simulink model "MAE547ComplianceControl"  (R2023b)
settings: Solver=VariableStepAuto  StartTime=0.0  StopTime=10  RelTol=1e-3
values from neighbouring files (symbols this model uses):
  Kd = diag([2 10 30 1 1 1])    [Parameters.m]
  Kp = diag([50 80 100 1 1 1])    [Parameters.m]
  l1 = param.l1    [B_Lagrangian.m]    (also in Manipulator.m = 0.4; Parameters.m)
  l2 = param.l2    [B_Lagrangian.m]    (also in Manipulator.m = 0.46; Parameters.m)
  l3 = param.l3    [B_Lagrangian.m]    (also in Manipulator.m = 0.15; Parameters.m)
  m1 = param.m1    [B_Lagrangian.m]    (also in Manipulator.m = 1)
  m2 = param.m2    [B_Lagrangian.m]    (also in Manipulator.m = 1)
  m3 = param.m3    [B_Lagrangian.m]    (also in Manipulator.m = 1)
  xd = Kinematics(q)    [Parameters.m]
undefined symbols (not defined in the file or in its folder): axis, wall
settings Model: Creator=andre  LastModifiedBy=zaner
settings SolverCC: AlgebraicLoopSolver=TrustRegion
settings DataIOCC: LimitDataPoints=on
settings DebuggingCC: UnconnectedInputMsg=warning  UnconnectedOutputMsg=warning  UnconnectedLineMsg=warning
settings ModelReferenceCC: EnableRefExpFcnMdlSchedulingChecks=on
settings RTWCC: DLArmComputeVersion=19.05

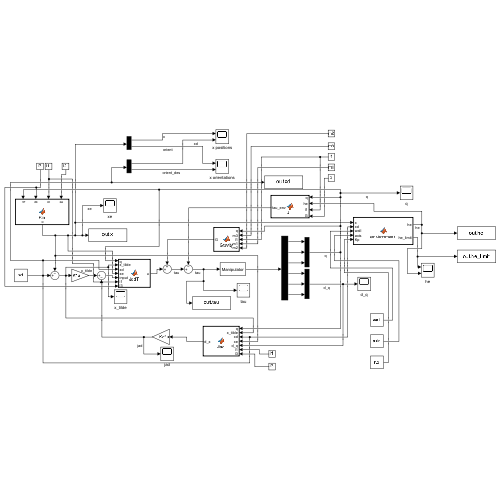
[thumbnail: Simulink's stored preview of the top-level diagram]
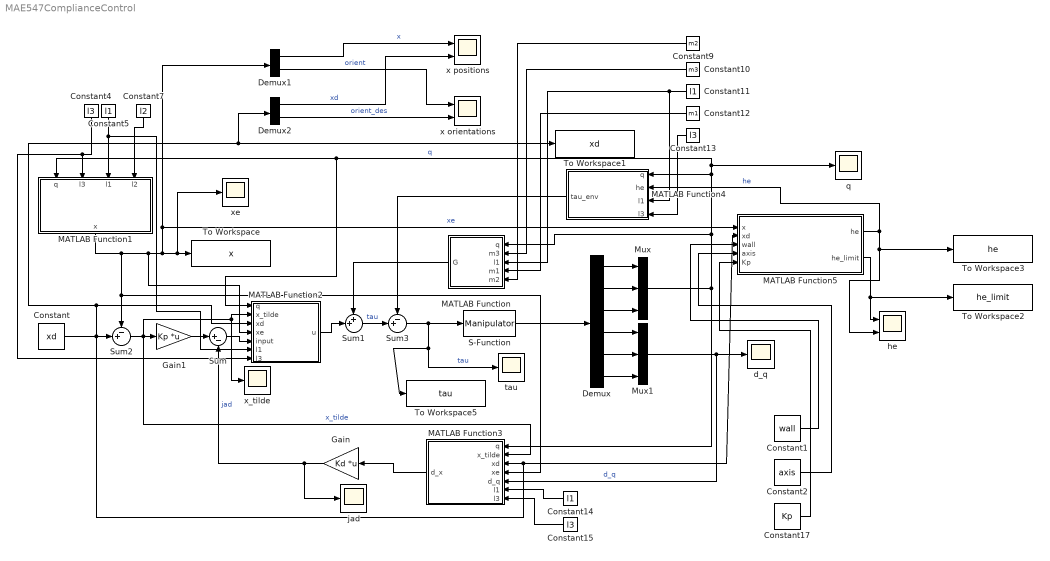
== system MAE547ComplianceControl ==
  Constant : Constant  Value=xd
  Constant1 : Constant  Value=wall
  Constant10 : Constant  Value=m3
  Constant11 : Constant  Value=l1
  Constant12 : Constant  Value=m1
  Constant13 : Constant  Value=l3
  Constant14 : Constant  Value=l1
  Constant15 : Constant  Value=l3
  Constant17 : Constant  Value=Kp
  Constant2 : Constant  Value=axis
  Constant4 : Constant  Value=l3
  Constant5 : Constant  Value=l1
  Constant7 : Constant  Value=l2
  Constant9 : Constant  Value=m2
  Demux : Demux  Outputs=6
  Demux1 : Demux  Outputs=2
  Demux2 : Demux  Outputs=2
  Gain : Gain  Gain=Kd  Multiplication=Matrix(K*u)
  Gain1 : Gain  Gain=Kp  Multiplication=Matrix(K*u)
  MATLAB Function : MATLAB Function  TreatAsAtomicUnit=on
  MATLAB Function1 : MATLAB Function  TreatAsAtomicUnit=on
  MATLAB Function2 : MATLAB Function  TreatAsAtomicUnit=on
  MATLAB Function3 : MATLAB Function  TreatAsAtomicUnit=on
  MATLAB Function4 : MATLAB Function  TreatAsAtomicUnit=on
  MATLAB Function5 : MATLAB Function  TreatAsAtomicUnit=on
  Mux : Mux  Inputs=3
  Mux1 : Mux  Inputs=3
  S-Function : S-Function  FunctionName=Manipulator  SFunctionDeploymentMode=off  EnableBusSupport=off
  Sum : Sum  Inputs=|+-
  Sum1 : Sum  Inputs=++|
  Sum2 : Sum  Inputs=-+|
  Sum3 : Sum  Inputs=-+|
  To Workspace : ToWorkspace  VariableName=x  SaveFormat=Timeseries  SampleTime=-1
  To Workspace1 : ToWorkspace  VariableName=xd  SaveFormat=Timeseries  SampleTime=-1
  To Workspace2 : ToWorkspace  VariableName=he_limit  SaveFormat=Timeseries  SampleTime=-1
  To Workspace3 : ToWorkspace  VariableName=he  SaveFormat=Timeseries  SampleTime=-1
  To Workspace5 : ToWorkspace  VariableName=tau  SaveFormat=Timeseries  SampleTime=-1
  d_q : Scope
  he : Scope  NumInputPorts=2
  jad : Scope
  q : Scope
  tau : Scope
  x orientations : Scope  NumInputPorts=2
  x positions : Scope  NumInputPorts=2
  x_tilde : Scope
  xe : Scope
  wires:
  Gain1/1 -> Sum/1
  Demux/3 -> Mux/3
  Demux/2 -> Mux/2
  Demux/1 -> Mux/1
  Demux/4 -> Mux1/1
  Demux/5 -> Mux1/2
  Demux/6 -> Mux1/3
  Mux/1 -> MATLAB Function3/1(q), MATLAB Function1/1(q), MATLAB Function2/1(q), q/1, MATLAB Function4/1(q), MATLAB Function/1(q)  "q"
  Gain/1 -> jad/1, Sum/2  "jad"
  Sum2/1 -> x_tilde/1, MATLAB Function2/2(x_tilde), MATLAB Function3/2(x_tilde), Gain1/1  "x_tilde"
  Mux1/1 -> MATLAB Function3/5(d_q), d_q/1  "d_q"
  Constant/1 -> MATLAB Function5/2(xd), MATLAB Function3/3(xd), Sum2/2, Demux2/1, To Workspace1/1, MATLAB Function2/3(xd)
  MATLAB Function1/1(x) -> MATLAB Function2/4(xe), Demux1/1, MATLAB Function5/1(x), xe/1, To Workspace/1, MATLAB Function3/4(xe), Sum2/1  "xe"
  MATLAB Function2/1(u) -> Sum1/2
  MATLAB Function3/1(d_x) -> Gain/1
  Demux1/1 -> x positions/1  "x"
  Demux2/1 -> x positions/2  "xd"
  Demux1/2 -> x orientations/1  "orient"
  Demux2/2 -> x orientations/2  "orient_des"
  Sum/1 -> MATLAB Function2/5(input)
  MATLAB Function5/1(he) -> MATLAB Function4/2(he), he/2, To Workspace3/1  "he"
  Sum3/1 -> S-Function/1, To Workspace5/1, tau/1  "tau"
  MATLAB Function5/2(he_limit) -> To Workspace2/1, he/1
  Sum1/1 -> Sum3/2  "tau"
  MATLAB Function/1(G) -> Sum1/1
  MATLAB Function4/1(tau_env) -> Sum3/1
  Constant1/1 -> MATLAB Function5/3(wall)
  Constant2/1 -> MATLAB Function5/4(axis)
  Constant7/1 -> MATLAB Function1/4(l2)
  Constant5/1 -> MATLAB Function2/6(l1), MATLAB Function1/3(l1)
  Constant4/1 -> MATLAB Function2/7(l3), MATLAB Function1/2(l3)
  Constant9/1 -> MATLAB Function/5(m2)
  Constant10/1 -> MATLAB Function/2(m3)
  Constant11/1 -> MATLAB Function4/3(l1), MATLAB Function/3(l1)
  Constant12/1 -> MATLAB Function/4(m1)
  Constant13/1 -> MATLAB Function4/4(l3)
  Constant14/1 -> MATLAB Function3/6(l1)
  Constant15/1 -> MATLAB Function3/7(l3)
  Constant17/1 -> MATLAB Function5/5(Kp)
  S-Function/1 -> Demux/1

== matlab function MAE547ComplianceControl/MATLAB Function1 ==
  data: q input; x output; l3 input; l1 input; l2 input
function x = Kin(q,l3,l1,l2)
    x = Kinematics(q,l3,l1,l2);
end

== matlab function MAE547ComplianceControl/MATLAB Function ==
  data: q input; m3 input; l1 input; m1 input; G output; m2 input
function G = Gravity(q,m3,l1,m1,m2)
   G = G_Lagrangian(q,m3,l1,m1,m2);
end

== matlab function MAE547ComplianceControl/MATLAB Function2 ==
  data: q input; x_tilde input; xd input; xe input; input input; u output; l1 input; l3 input
function u = JadT(q, x_tilde, xd,xe, input,l1,l3)
    Ja = getJad(q, x_tilde, xd, xe,l1,l3);
    u = Ja' * input;
end

== matlab function MAE547ComplianceControl/MATLAB Function3 ==
  data: q input; x_tilde input; xd input; xe input; d_q input; d_x output; l1 input; l3 input
function d_x = Jad(q, x_tilde, xd, xe, d_q, l1, l3)
    Ja = getJad(q, x_tilde, xd, xe, l1, l3);
    d_x = Ja * d_q;
end

== matlab function MAE547ComplianceControl/MATLAB Function4 ==
  data: q input; he input; tau_env output; l1 input; l3 input
function tau_env = JT(q, he,l1,l3)
    tau_env = Jacobian(q,l1,l3)' * he;
end

== matlab function MAE547ComplianceControl/MATLAB Function5 ==
  data: x input; he output; xd input; he_limit output; wall input; axis input; Kp input
function [he, he_limit] = environment(x, xd,wall,axis,Kp)
    K = 200*diag([1 1 1 1 1 1]); 
    if x(axis) >= wall 

        % set up the rest position frame
        xr = zeros(6,1);
        xr(axis) = wall;

        xe = zeros(6,1);
        xe(axis) = x(axis);

        he = K * (xe - xr);
        dx_rd = zeros(6,1);
        dx_rd(axis) = xd(axis) - xr(axis);
        % At the limit
        he_limit =  K/(eye(6) + K / Kp) * dx_rd;
    else
        he = zeros(6,1);
        he_limit = zeros(6,1);
    end
end
